simulink model "Gimbal_Model"  (R2024b)
settings: Solver=ode5  StartTime=0.0  StopTime=inf  RelTol=1e-3
undefined symbols (not defined in the file): Baz, Bel, Bm, Jaz, Jel, Jm, K_cf, Ke, Km, L, R, Sim3dSensor, Standard_Devices, Tpade, UDP_Protocol
libraries: slpidlib x2, simulink_extras x2, sldrtlib x2, visionsinks x1, simulink x1, sim3dcameralib x1, sim3dlib x1, sim3dautolib x1
settings Model: Creator=The MathWorks, Inc.  LastModifiedBy=lucas
settings OptimizationCC: ReuseModelBlockBuffer=off
settings DebuggingCC: SubsystemReferenceDiagnosticForUnitTest=warning
settings HardwareCC: ProdBitPerLong=64  ProdHWDeviceType=Intel->x86-64 (Linux 64)
settings RTWCC: Description=Simulink Desktop Real-Time  SystemTargetFile=sldrt.tlc  TemplateMakefile=sldrt.tmf  RTWCompilerOptimization=on  GPUComputeCapability=3.5
settings CodeAppCC: MaxIdLength=95
settings SimulinkDesktopRealTimeCC: TargetLibSuffix=_sldrt.a  TargetPreCompLibLocation=C:\Program Files\MATLAB\R2024b\toolbox\sldrt\lib\win64  ParMdlRefBuildCompliant=on

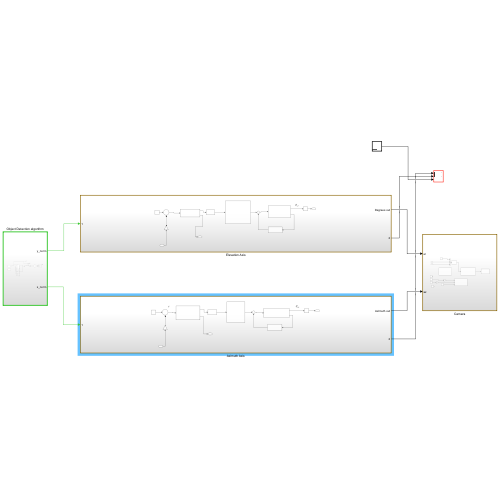
[thumbnail: Simulink's stored preview of the top-level diagram]
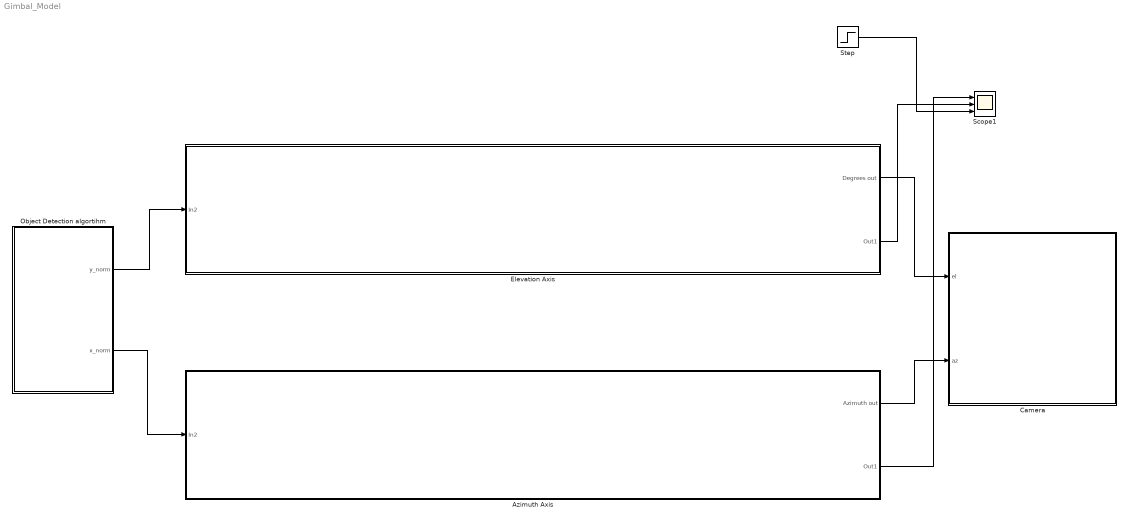
== system Gimbal_Model ==
  Azimuth Axis : Subsystem
  Camera : Subsystem
  Elevation Axis : Subsystem
  Object Detection algortihm : Subsystem  TreatAsAtomicUnit=on
  Scope1 : Scope  NumInputPorts=3
  Step : Step  After=0  SampleTime=0
  wires:
  Elevation Axis/1(Degrees out) -> Camera/1(el)
  Azimuth Axis/1(Azimuth out) -> Camera/2(az)
  Object Detection algortihm/1(y_norm) -> Elevation Axis/1(In2)
  Object Detection algortihm/2(x_norm) -> Azimuth Axis/1(In2)
  Step/1 -> Scope1/3
  Elevation Axis/2(Out1) -> Scope1/2
  Azimuth Axis/2(Out1) -> Scope1/1

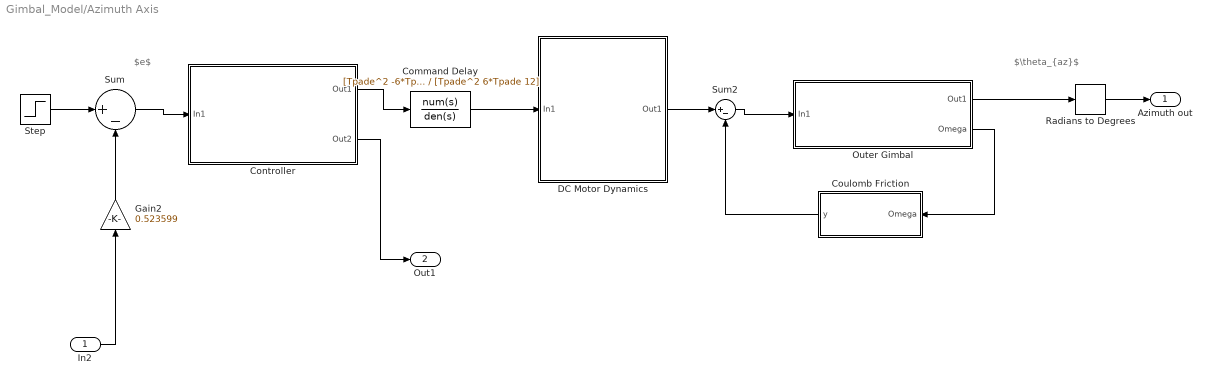
== system Gimbal_Model/Azimuth Axis ==
  note: $e$
  note: $\theta_{az}$
  In2 : Inport
  Command Delay : TransferFcn  Numerator=[Tpade^2 -6*Tpade 12]  Denominator=[Tpade^2 6*Tpade 12]
  Controller : Subsystem
  Coulomb Friction : Subsystem
  DC Motor Dynamics : Subsystem
  Gain2 : Gain  Gain=0.523599
  Outer Gimbal : Subsystem
  Radians to Degrees : simulink_extras/Transformations/Radians to Degrees
  Step : Step  Time=0  After=0  SampleTime=0
  Sum : Sum  Inputs=|+-
  Sum2 : Sum  Inputs=|+-
  Azimuth out : Outport
  Out1 : Outport  Port=2
  wires:
  Sum2/1 -> Outer Gimbal/1(In1)
  Step/1 -> Sum/1
  In2/1 -> Gain2/1
  Radians to Degrees/1 -> Azimuth out/1
  Command Delay/1 -> DC Motor Dynamics/1(In1)
  DC Motor Dynamics/1(Out1) -> Sum2/1
  Outer Gimbal/1(Out1) -> Radians to Degrees/1
  Sum/1 -> Controller/1(In1)
  Controller/1(Out1) -> Command Delay/1
  Coulomb Friction/1(y) -> Sum2/2
  Outer Gimbal/2(Omega) -> Coulomb Friction/1(Omega)
  Gain2/1 -> Sum/2
  Controller/2(Out2) -> Out1/1

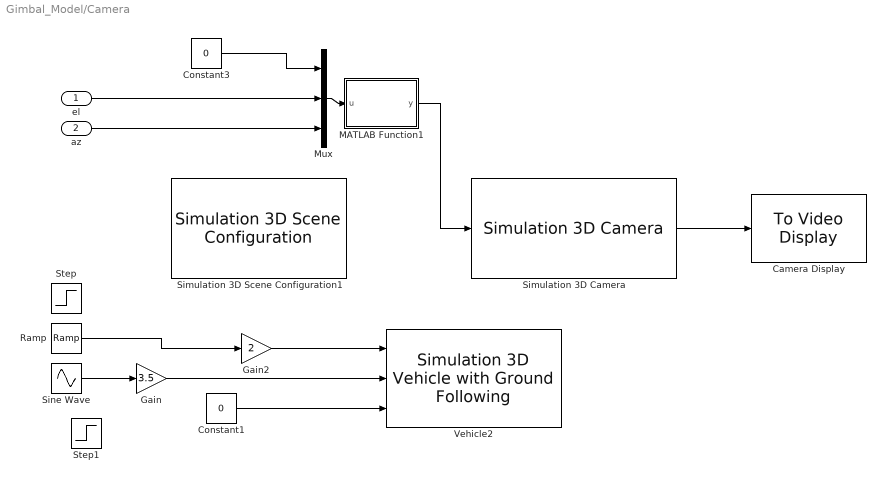
== system Gimbal_Model/Camera ==
  el : Inport
  az : Inport  Port=2
  Camera Display : visionsinks/To Video Display  windowSizeMode=Normal  openAtMdlStart=on  fullScreen=off  videoWindowX=536805376  videoWindowY=536805376  saveWindowSize=off  videoWindowWidth=822  videoWindowHeight=448  inputColorFormat=RGB  inputType=Obsolete  imagePorts=One multidimensional signal  OutputDevice=On-screen video monitor  dataOrg=Column-major  isWindowOpen=off
  Constant1 : Constant  Value=0
  Constant3 : Constant  Value=0
  Gain : Gain  Gain=3.5
  Gain2 : Gain  Gain=2
  MATLAB Function1 : MATLAB Function  TreatAsAtomicUnit=on
  Mux : Mux  Inputs=3
  Ramp : simulink/Sources/Ramp  slope=3  start=0  InitialOutput=0
  Simulation 3D Camera : sim3dcameralib/Simulation 3D Camera  Priority=1  sensorTag=Sim3dSensor�  sensorId=3  sensorName=Sim3dSensor�  vehTagList={'Scene Origin';'SimulinkVehicle2'}  vehTag=Scene Origin  mountLoc=Origin  offsetFlag=on  tmountOffset=[0, 0, 20]  extTmount=off  rmountOffset=[0,45,0]  extRmount=on  FocalLength=[1109, 1109]  OpticalCenter=[640, 360]  ImageSize=[720, 1280]  RadialDistortion=[0, 0]  TangentialDistortion=[0, 0]  SensorSkew=0  DepthOutportEnabled=off  SemanticOutportEnabled=off  TransformOutportEnabled=off  SampleTime=1/60  mountPoint=[0 0 20]  mountOrientation=[0 -45 0]  aMode=3  ID=3
      settings: LibrarySourceBlock=drivingsim3d/Simulation 3D Camera
  Simulation 3D Scene Configuration1 : sim3dlib/Simulation 3D Scene Configuration  Priority=0  ProjectFormat=Default Scenes  SceneDesc=Straight road  ProjectName=C:\Program Files\MATLAB\R2024b\toolbox\shared\sim3d_projects\automotive_project_windows\UE\WindowsNoEditor\VehicleSimulation.exe  ScenePath=/Game/Maps/HwStrght  RoadRunnerProjectPath=./Data/sim3dRoad.fbx  EnableOpenDRIVE=off  vehTagList={'Custom';'Scene Origin';'SimulinkVehicle1';'SimulinkVehicle2'}  vehTag=SimulinkVehicle2  FreeCameraInitialTranslation=[0, 0, 0]  FreeCameraDefaultInitialTranslation=[-6, 0, 2]  FreeCameraInitialRotation=[0, 0, 0]  FreeCameraDefaultInitialRotation=[0, -15, 0]  OpVisEn=off  Ts=1/60  EnableWindow=off  EnableRemoteAccess=off  EnableWeather=off  SunAzimuth=90  SunAltitude=40.0  EnableGeospatialSun=off  Latitude=0  Longitude=0  Date=2023-01-01  Time=10:30:00  GeoTimeZone=-5.0  SunDaylightSaving=off  wind=1  clouds=10  EnableVolumetricClouds=off  CloudCoverage=0  CloudAltitude=6  fog=0  rain=0  RaindropsEffect=off  SnowDensity=0  EnableGeospatial=off  UseTrueOrigin=off  OriginHeight=200  OriginLatitude=40.744652  OriginLongitude=-73.988864  MapStyle=Aerial  AdditionalAssetIDs=[]  UseAdvancedSunSky=off  SolarTime=11  TimeZone=-5  Day=21  Month=9  Year=2022  UseDaylightSavingTime=on  DSTStartDay=10  DSTStartMonth=3  DSTEndDay=3  DSTEndMonth=11  DSTSwitchHour=2  sensorTag=MainCamera2  sensorId=2  sensorName=MainCamera2  mountLoc=Origin  offsetFlag=off  tmountOffset=[0, 0, 0]  rmountOffset=[0, 0, 0]  HorizontalResolution=1280  VerticalResolution=720  HorizontalFOV=60  mountPoint=[0 0 0]  mountOrientation=[0 0 0]  aMode=3  ID=2  GeoTrigger=Inactive
      settings: LibrarySourceBlock=drivingsim3d/Simulation 3D Scene Configuration
  Sine Wave : Sin  Amplitude=3  Frequency=0.5*pi  SampleTime=0
  Step : Step  Time=10  After=16  SampleTime=0
  Step1 : Step  Time=10  After=2.5  SampleTime=0
  Vehicle2 : sim3dautolib/Simulation 3D Vehicle with Ground Following  Priority=-1  PassVehMesh=Muscle car  MeshPath=/MathWorksAutomotiveContent/Vehicles/Muscle/Meshes/SK_MuscleCar.SK_MuscleCar  TrackWidth=1.9  WheelBase=3  WheelRadius=0.35  VehColor=Red  InitialPos=[10, -1.5, 0]  InitialRot=[0, 0, 0]  ActorName=SimulinkVehicle2  SampleTime=-1  ActorType=SimulinkVehicle  ID=2  aMode=3  ActorTag=SimulinkVehicle2  CoordinateScheme=ISO  VehLightsControl=off  HeadlightColor=[ 1, 1, 1 ]  HighBeamIntensity=100000  LowBeamIntensity=60000  HighBeamConeAngle=70  LowBeamConeAngle=70  LeftHeadlightOrientation=[ 0, 0 ]  RightHeadlightOrientation=[ 0, 0 ]  BrakelightIntensity=500  ReverselightIntensity=500  SignallightIntensity=500  SignallightPeriod=1  SignalPulseWidth=50  TransformOutportEnabled=off
      settings: LibrarySourceBlock=drivingsim3d/Simulation 3D Vehicle with Ground Following
  wires:
  MATLAB Function1/1(y) -> Simulation 3D Camera/1
  Gain/1 -> Vehicle2/2
  Gain2/1 -> Vehicle2/1
  Mux/1 -> MATLAB Function1/1(u)
  Constant1/1 -> Vehicle2/3
  Constant3/1 -> Mux/1
  Simulation 3D Camera/1 -> Camera Display/1
  el/1 -> Mux/2
  az/1 -> Mux/3
  Sine Wave/1 -> Gain/1
  Ramp/1 -> Gain2/1

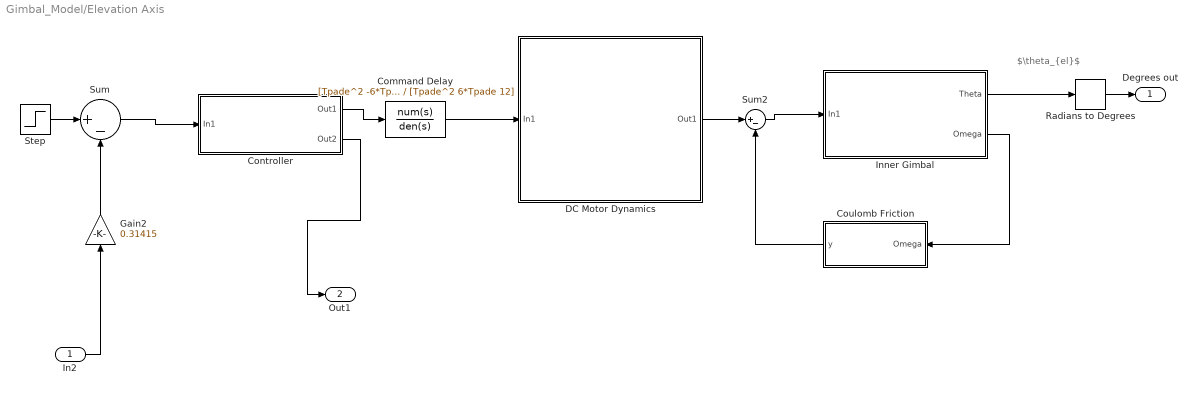
== system Gimbal_Model/Elevation Axis ==
  note: $\theta_{el}$
  In2 : Inport
  Command Delay : TransferFcn  Numerator=[Tpade^2 -6*Tpade 12]  Denominator=[Tpade^2 6*Tpade 12]
  Controller : Subsystem
  Coulomb Friction : Subsystem
  DC Motor Dynamics : Subsystem
  Gain2 : Gain  Gain=0.31415
  Inner Gimbal : Subsystem
  Radians to Degrees : simulink_extras/Transformations/Radians to Degrees
  Step : Step  Time=0  After=0  SampleTime=0
  Sum : Sum  Inputs=|+-
  Sum2 : Sum  Inputs=|+-
  Degrees out : Outport
  Out1 : Outport  Port=2
  wires:
  In2/1 -> Gain2/1
  Radians to Degrees/1 -> Degrees out/1
  Sum2/1 -> Inner Gimbal/1(In1)
  Command Delay/1 -> DC Motor Dynamics/1(In1)
  DC Motor Dynamics/1(Out1) -> Sum2/1
  Inner Gimbal/1(Theta) -> Radians to Degrees/1
  Sum/1 -> Controller/1(In1)
  Controller/1(Out1) -> Command Delay/1
  Inner Gimbal/2(Omega) -> Coulomb Friction/1(Omega)
  Coulomb Friction/1(y) -> Sum2/2
  Gain2/1 -> Sum/2
  Step/1 -> Sum/1
  Controller/2(Out2) -> Out1/1

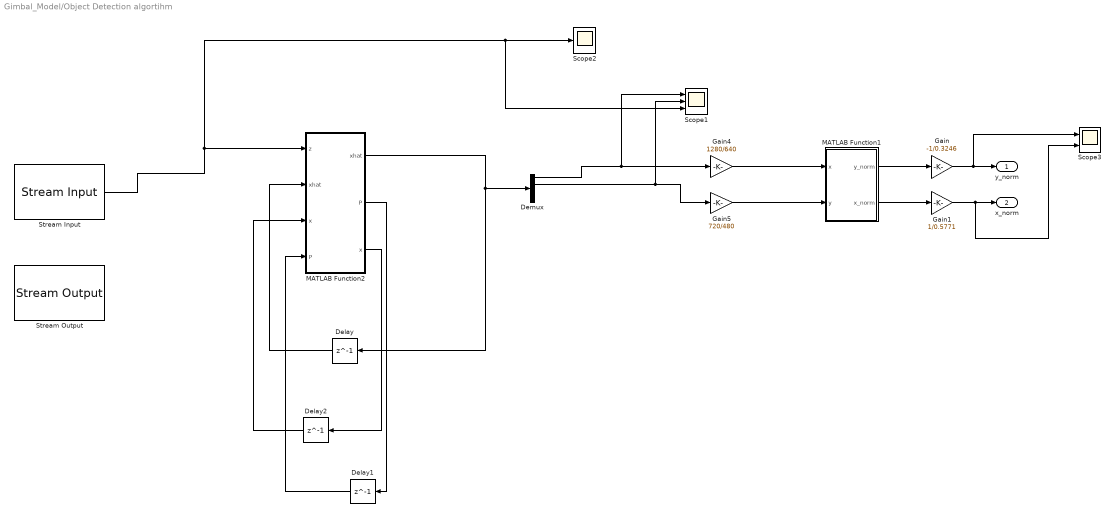
== system Gimbal_Model/Object Detection algortihm ==
  Delay : Delay  DelayLength=1  InitialCondition=[320;240;0;0]
  Delay1 : Delay  DelayLength=1
  Delay2 : Delay  DelayLength=1  InitialCondition=0
  Demux : Demux
  Gain : Gain  Gain=-1/0.3246
  Gain1 : Gain  Gain=1/0.5771
  Gain4 : Gain  Gain=1280/640
  Gain5 : Gain  Gain=720/480
  MATLAB Function1 : MATLAB Function  TreatAsAtomicUnit=on
  MATLAB Function2 : MATLAB Function  TreatAsAtomicUnit=on
  Scope1 : Scope  NumInputPorts=3
  Scope2 : Scope
  Scope3 : Scope  NumInputPorts=2
  Stream Input : sldrtlib/Stream Input  ExecutionOrder=First  SampleTime=1/10000  MaxMissedTicks=inf  ShowMissedTicks=off  YieldWhenWaiting=on  DrvName=Standard_Devices/UDP_Protocol  DrvAddress=50924  DrvOptions=[0 16385 0 0 0 0 0 0 0 0 0 0 0 0 0 0 0 0 0 0 0 0 0 0 0 0 0 0 0 0 0 0 0 0 0 0 0 0 0 0 0 0 0 0 0 0 0 0 0 0 0 0 0 0 0 0 0 0 0 0 0 0 0 0 0 0 0 0 0 0 0 0 0 0 0 0 0 0 0 0 0 0 0 0 0 0 0 0 0 0 0 0 0 0 0 0 0 0 0 0 0 0 0 0 0 0 0 0 0 0 0 0 0 0 0 0 0 0 0 0 0 0 0 0 0 0 0 0 0 0 0 0 0 0 0 0 0 0 0 0 0 0 0 0 0 0 0 0 0 0 0 0 0 0 0 0 0 0 0 0 0 0 0 0 0 0 0 0 0 0 0 0 0 0 0 0 0 0 0 0 0 0 0 0 0 0 0 0 0 0 0 0 0 0 0 0 0 0 0 0 0 0 0 0 0 0 0 0 0 0 0 0 0 0 0 0 0 0 0 0 0 0 0 0 0 0 0 0 0 0 0 0 0 0 0 0 0 0 0 0 0 0 0 0 0 0 0 0 0 0 0 0 0 0 0 0]  DataTypes={'2*double'}  FormatString='%f %f '  Terminator={'\n'}  ShowReady=off  ShowError=off
      settings: AttributesFormatString=UDP Protocol [50924]
  Stream Output : sldrtlib/Stream Output  SampleTime=1/10000  MaxMissedTicks=inf  ShowMissedTicks=off  YieldWhenWaiting=on  DrvName=Standard_Devices/UDP_Protocol  DrvAddress=50924  DrvOptions=[0 16385 0 0 0 0 0 0 0 0 0 0 0 0 0 0 0 0 0 0 0 0 0 0 0 0 0 0 0 0 0 0 0 0 0 0 0 0 0 0 0 0 0 0 0 0 0 0 0 0 0 0 0 0 0 0 0 0 0 0 0 0 0 0 0 0 0 0 0 0 0 0 0 0 0 0 0 0 0 0 0 0 0 0 0 0 0 0 0 0 0 0 0 0 0 0 0 0 0 0 0 0 0 0 0 0 0 0 0 0 0 0 0 0 0 0 0 0 0 0 0 0 0 0 0 0 0 0 0 0 0 0 0 0 0 0 0 0 0 0 0 0 0 0 0 0 0 0 0 0 0 0 0 0 0 0 0 0 0 0 0 0 0 0 0 0 0 0 0 0 0 0 0 0 0 0 0 0 0 0 0 0 0 0 0 0 0 0 0 0 0 0 0 0 0 0 0 0 0 0 0 0 0 0 0 0 0 0 0 0 0 0 0 0 0 0 0 0 0 0 0 0 0 0 0 0 0 0 0 0 0 0 0 0 0 0 0 0 0 0 0 0 0 0 0 0 0 0 0 0 0 0 0 0 0 0]  PortSizes=[1]  FormatString='%f'  ShowReady=off  ShowError=off  InitialValue=[]  FinalValue=[]
      settings: AttributesFormatString=UDP Protocol [50924]
  y_norm : Outport
  x_norm : Outport  Port=2
  wires:
  MATLAB Function2/2(P) -> Delay1/1
  MATLAB Function2/1(xhat) -> Delay/1, Demux/1
  Delay/1 -> MATLAB Function2/2("xhat ")
  Delay1/1 -> MATLAB Function2/4("P ")
  Demux/1 -> Scope1/1, Gain4/1
  Demux/2 -> Scope1/2, Gain5/1
  MATLAB Function1/1(y_norm) -> Gain/1
  MATLAB Function1/2(x_norm) -> Gain1/1
  Gain/1 -> Scope3/1, y_norm/1
  Gain1/1 -> Scope3/2, x_norm/1
  Gain5/1 -> MATLAB Function1/2(y)
  Gain4/1 -> MATLAB Function1/1(x)
  MATLAB Function2/3(x) -> Delay2/1
  Delay2/1 -> MATLAB Function2/3("x ")
  Stream Input/1 -> MATLAB Function2/1(z), Scope1/3, Scope2/1

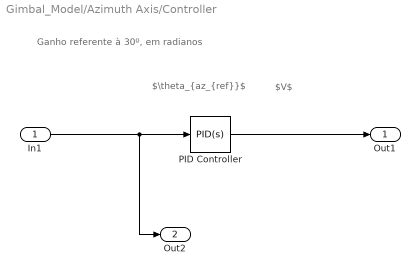
== system Gimbal_Model/Azimuth Axis/Controller ==
  note: Ganho referente à 30º, em radianos
  note: $\theta_{az_{ref}}$
  note: $V$
  In1 : Inport
  PID Controller : slpidlib/PID Controller  Controller=PID  Form=Parallel  TimeDomain=Continuous-time  UseExternalTs=off  SampleTime=-1  IntegratorMethod=Forward Euler  FilterMethod=Forward Euler  ControllerParametersSource=internal  P=0.5  I=0.2  UseKiTs=off  D=0.45  UseExternalDerivativeSource=off  N=100  UseFilter=on  TunerSelectOption=Transfer Function Based (PID Tuner App)  InitialConditionSource=internal  InitialConditionForIntegrator=0  InitialConditionForFilter=0  DifferentiatorICPrevScaledInput=0  ExternalReset=none  TrackingMode=off  Kt=1  LimitOutput=off  SatLimitsSource=internal  UpperSaturationLimit=inf  LowerSaturationLimit=-inf  LinearizeAsGain=on  AntiWindupMode=none  Kb=1  LimitIntegrator=off  UpperIntegratorSaturationLimit=inf  LowerIntegratorSaturationLimit=-inf  POutMin=[]  POutMax=[]  IOutMin=[]  IOutMax=[]  DOutMin=[]  DOutMax=[]  NOutMin=[]  NOutMax=[]  SumOutMin=[]  SumOutMax=[]  SaturationOutMin=[]  SaturationOutMax=[]  PParamMin=[]  PParamMax=[]  IParamMin=[]  IParamMax=[]  DParamMin=[]  DParamMax=[]  NParamMin=[]  NParamMax=[]  KbParamMin=[]  KbParamMax=[]  KtParamMin=[]  KtParamMax=[]  KbOutMin=[]  KbOutMax=[]  KtOutMin=[]  KtOutMax=[]  IntegratorOutMin=[]  IntegratorOutMax=[]  FilterOutMin=[]  FilterOutMax=[]  SumI1OutMin=[]  SumI1OutMax=[]  SumI2OutMin=[]  SumI2OutMax=[]  SumI3OutMin=[]  SumI3OutMax=[]  SumI4OutMin=[]  SumI4OutMax=[]  SumDOutMin=[]  SumDOutMax=[]  DifferentiatorOutMin=[]  DifferentiatorOutMax=[]  FilterDiffOutCoefMin=[]  FilterDiffOutCoefMax=[]  ReciprocalOutMin=[]  ReciprocalOutMax=[]  SumDenOutMin=[]  SumDenOutMax=[]  SumNumOutMin=[]  SumNumOutMax=[]  DivideOutMin=[]  DivideOutMax=[]  UdiffTsProdOutMin=[]  UdiffTsProdOutMax=[]  NTsProdOutMin=[]  NTsProdOutMax=[]  UintegralTsProdOutMin=[]  UintegralTsProdOutMax=[]  UngainTsProdOutMin=[]  UngainTsProdOutMax=[]  ClampingZeroOutDataTypeStr=Inherit: Inherit via back propagation  ClampingZeroOutMin=[]  ClampingZeroOutMax=[]  FilterDenConstantOutDataTypeStr=Inherit: Inherit via back propagation  FilterDenConstantOutMin=[]  FilterDenConstantOutMax=[]  PCopyOutDataTypeStr=Inherit: Inherit via back propagation  PCopyOutMin=[]  PCopyOutMax=[]  NCopyOutDataTypeStr=Inherit: Inherit via back propagation  NCopyOutMin=[]  NCopyOutMax=[]  IntegratorContinuousStateAttributes=''  IntegratorStateMustResolveToSignalObject=off  IntegratorRTWStateStorageClass=Auto  FilterContinuousStateAttributes=''  FilterStateMustResolveToSignalObject=off  FilterRTWStateStorageClass=Auto  ParallelPVariant=InternalParameters  IdealPVariant=Disabled  IVariant=InternalParameters  DVariant=InternalParameters  IntegratorVariant=Continuous  SatVariant=Disabled  AWVariant=Passthrough  PCopyVariant=Disabled  TRVariant=Disabled  FdbkBlocksVariant=Forward  IdealPFdbkVariant=Disabled  SatFdbkVariant=Disabled  DerivativeFilterVariant=ContFilter  NVariant=InternalParameters  NCopyVariant=Disabled  FilterICVariant=InternalICsFilter  IntegratorICVariant=InternalICs  ExternalResetVariant=Disabled  TRSumVariant=Passthrough  SumFdbkVariant=Disabled  SumVariant=Sum_PID  TsampFilterVariant=InternalTs  TsampNgainVariant=Passthrough  TsampIntegralVariant=Disabled_SignalSpec  ExternalSaturationOutDataTypeStr=Inherit: Same as second input  DerivativeSourceVariant=ErrorSignal  PreIntVariant=InternalPreInt
  Out1 : Outport
  Out2 : Outport  Port=2
  wires:
  PID Controller/1 -> Out1/1
  In1/1 -> Out2/1, PID Controller/1

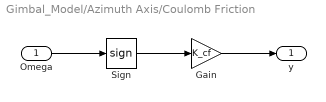
== system Gimbal_Model/Azimuth Axis/Coulomb Friction ==
  Omega : Inport
  Gain : Gain  Gain=K_cf
  Sign : Signum
  y : Outport
  wires:
  Omega/1 -> Sign/1
  Gain/1 -> y/1
  Sign/1 -> Gain/1

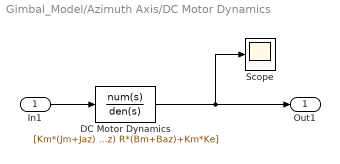
== system Gimbal_Model/Azimuth Axis/DC Motor Dynamics ==
  In1 : Inport
  DC Motor Dynamics : TransferFcn  Numerator=[Km*(Jm+Jaz) Km*(Baz+Bm)]  Denominator=[L*(Jm+Jaz) R*(Jm+Jaz)+L*(Bm+Baz) R*(Bm+Baz)+Km*Ke]
  Scope : Scope
  Out1 : Outport
  wires:
  In1/1 -> DC Motor Dynamics/1
  DC Motor Dynamics/1 -> Scope/1, Out1/1

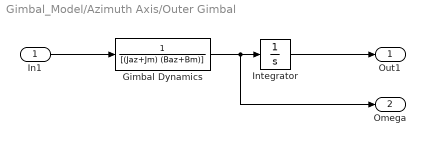
== system Gimbal_Model/Azimuth Axis/Outer Gimbal ==
  In1 : Inport
  Gimbal Dynamics : TransferFcn  Denominator=[(Jaz+Jm) (Baz+Bm)]
  Integrator : Integrator
  Out1 : Outport
  Omega : Outport  Port=2
  wires:
  Integrator/1 -> Out1/1
  In1/1 -> Gimbal Dynamics/1
  Gimbal Dynamics/1 -> Omega/1, Integrator/1

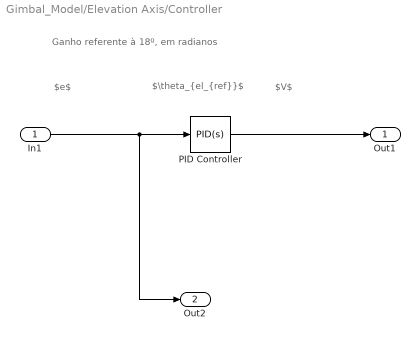
== system Gimbal_Model/Elevation Axis/Controller ==
  note: Ganho referente à 18º, em radianos
  note: $\theta_{el_{ref}}$
  note: $e$
  note: $V$
  In1 : Inport
  PID Controller : slpidlib/PID Controller  Controller=PID  Form=Parallel  TimeDomain=Continuous-time  UseExternalTs=off  SampleTime=-1  IntegratorMethod=Forward Euler  FilterMethod=Forward Euler  ControllerParametersSource=internal  P=0.5  I=0.15  UseKiTs=off  D=0.5  UseExternalDerivativeSource=off  N=100  UseFilter=on  TunerSelectOption=Transfer Function Based (PID Tuner App)  InitialConditionSource=internal  InitialConditionForIntegrator=0  InitialConditionForFilter=0  DifferentiatorICPrevScaledInput=0  ExternalReset=none  TrackingMode=off  Kt=1  LimitOutput=off  SatLimitsSource=internal  UpperSaturationLimit=inf  LowerSaturationLimit=-inf  LinearizeAsGain=on  AntiWindupMode=none  Kb=1  LimitIntegrator=off  UpperIntegratorSaturationLimit=inf  LowerIntegratorSaturationLimit=-inf  POutMin=[]  POutMax=[]  IOutMin=[]  IOutMax=[]  DOutMin=[]  DOutMax=[]  NOutMin=[]  NOutMax=[]  SumOutMin=[]  SumOutMax=[]  SaturationOutMin=[]  SaturationOutMax=[]  PParamMin=[]  PParamMax=[]  IParamMin=[]  IParamMax=[]  DParamMin=[]  DParamMax=[]  NParamMin=[]  NParamMax=[]  KbParamMin=[]  KbParamMax=[]  KtParamMin=[]  KtParamMax=[]  KbOutMin=[]  KbOutMax=[]  KtOutMin=[]  KtOutMax=[]  IntegratorOutMin=[]  IntegratorOutMax=[]  FilterOutMin=[]  FilterOutMax=[]  SumI1OutMin=[]  SumI1OutMax=[]  SumI2OutMin=[]  SumI2OutMax=[]  SumI3OutMin=[]  SumI3OutMax=[]  SumI4OutMin=[]  SumI4OutMax=[]  SumDOutMin=[]  SumDOutMax=[]  DifferentiatorOutMin=[]  DifferentiatorOutMax=[]  FilterDiffOutCoefMin=[]  FilterDiffOutCoefMax=[]  ReciprocalOutMin=[]  ReciprocalOutMax=[]  SumDenOutMin=[]  SumDenOutMax=[]  SumNumOutMin=[]  SumNumOutMax=[]  DivideOutMin=[]  DivideOutMax=[]  UdiffTsProdOutMin=[]  UdiffTsProdOutMax=[]  NTsProdOutMin=[]  NTsProdOutMax=[]  UintegralTsProdOutMin=[]  UintegralTsProdOutMax=[]  UngainTsProdOutMin=[]  UngainTsProdOutMax=[]  ClampingZeroOutDataTypeStr=Inherit: Inherit via back propagation  ClampingZeroOutMin=[]  ClampingZeroOutMax=[]  FilterDenConstantOutDataTypeStr=Inherit: Inherit via back propagation  FilterDenConstantOutMin=[]  FilterDenConstantOutMax=[]  PCopyOutDataTypeStr=Inherit: Inherit via back propagation  PCopyOutMin=[]  PCopyOutMax=[]  NCopyOutDataTypeStr=Inherit: Inherit via back propagation  NCopyOutMin=[]  NCopyOutMax=[]  IntegratorContinuousStateAttributes=''  IntegratorStateMustResolveToSignalObject=off  IntegratorRTWStateStorageClass=Auto  FilterContinuousStateAttributes=''  FilterStateMustResolveToSignalObject=off  FilterRTWStateStorageClass=Auto  ParallelPVariant=InternalParameters  IdealPVariant=Disabled  IVariant=InternalParameters  DVariant=InternalParameters  IntegratorVariant=Continuous  SatVariant=Disabled  AWVariant=Passthrough  PCopyVariant=Disabled  TRVariant=Disabled  FdbkBlocksVariant=Forward  IdealPFdbkVariant=Disabled  SatFdbkVariant=Disabled  DerivativeFilterVariant=ContFilter  NVariant=InternalParameters  NCopyVariant=Disabled  FilterICVariant=InternalICsFilter  IntegratorICVariant=InternalICs  ExternalResetVariant=Disabled  TRSumVariant=Passthrough  SumFdbkVariant=Disabled  SumVariant=Sum_PID  TsampFilterVariant=InternalTs  TsampNgainVariant=Passthrough  TsampIntegralVariant=Disabled_SignalSpec  ExternalSaturationOutDataTypeStr=Inherit: Same as second input  DerivativeSourceVariant=ErrorSignal  PreIntVariant=InternalPreInt
  Out1 : Outport
  Out2 : Outport  Port=2
  wires:
  In1/1 -> Out2/1, PID Controller/1
  PID Controller/1 -> Out1/1

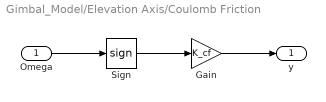
== system Gimbal_Model/Elevation Axis/Coulomb Friction ==
  Omega : Inport
  Gain : Gain  Gain=K_cf
  Sign : Signum
  y : Outport
  wires:
  Omega/1 -> Sign/1
  Gain/1 -> y/1
  Sign/1 -> Gain/1

== system Gimbal_Model/Elevation Axis/DC Motor Dynamics ==
  In1 : Inport
  DC Motor Dynamics : TransferFcn  Numerator=[Km*(Jm+Jel) Km*(Bel+Bm)]  Denominator=[L*(Jm+Jel) R*(Jm+Jel)+L*(Bm+Bel) R*(Bm+Bel)+Km*Ke]
  Out1 : Outport
  wires:
  In1/1 -> DC Motor Dynamics/1
  DC Motor Dynamics/1 -> Out1/1

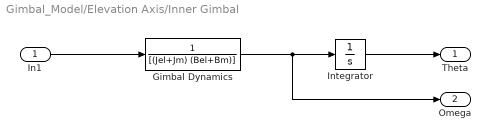
== system Gimbal_Model/Elevation Axis/Inner Gimbal ==
  In1 : Inport
  Gimbal Dynamics : TransferFcn  Denominator=[(Jel+Jm) (Bel+Bm)]
  Integrator : Integrator
  Theta : Outport
  Omega : Outport  Port=2
  wires:
  Integrator/1 -> Theta/1
  Gimbal Dynamics/1 -> Omega/1, Integrator/1
  In1/1 -> Gimbal Dynamics/1

== matlab function Gimbal_Model/Camera/MATLAB Function1 ==
  data: u input; y output
function y = fcn(u)

y = transpose(u);

== matlab function Gimbal_Model/Object Detection algortihm/MATLAB Function2 ==
  data: z input; xhat output size=[4,1]; P output size=[4, 4]; xhat input size=[4,1]; x input size=[4,1]; P input size=[4, 4]; x output
%Filtro de Kalman
function [xhat, P, x]= fcn(z,xhat,x,P)
T = 0.002;
sigma_acc = 4; %Desvio Padrão da aceleração 
sigma_cam = 1000; %Desvio Padrão do modelo de observação
u = transpose([1 1]); %Vetor de entrada.

A = [1 0 T 0
     0 1 0 T
     0 0 1 0
     0 0 0 1];

B = [T^2/2 0
     0 T^2/2
     T 0
     0 T];

C = [1 0 0 0
     0 1 0 0];

M = [sigma_acc^2 0
     0 sigma_acc^2];

Q = B*M*transpose(B);

R = [sigma_cam^2 0
     0 sigma_cam^2];

%Sistema físico
x = A*x + B*u; 

%Prediction step
xhat = A*xhat; %Estimativa
P = A*P*transpose(A) + Q; %Covariancia

%Filtering step 
K = P*transpose(C)*inv(R + C*P*transpose(C)); %Atualiza o ganho de Kalman
xhat = xhat + K*((z - C*xhat)); %Filtragem
P = P - K*C*P; %Atualiza a Covariancia

== matlab function Gimbal_Model/Object Detection algortihm/MATLAB Function1 ==
  data: y_norm output; x input; x_norm output; y input
function [y_norm, x_norm] = fcn(x, y)

K_camera_inv = [0.0009         0   -0.5771
                0    0.0009   -0.3246
                0         0    1.0000];
vec_pixel = [x;y;1];

vec_norm = K_camera_inv*vec_pixel;

x_norm = vec_norm(1);
y_norm = vec_norm(2);
